simulink model "lab2_aula"  (R2024b)
settings: Solver=VariableStepAuto  StartTime=0.0  StopTime=10000  MaxStep=1  RelTol=1e-3
settings Model: Creator=Diego Regruto  LastModifiedBy=stefa
settings RTWCC: GPUComputeCapability=3.5

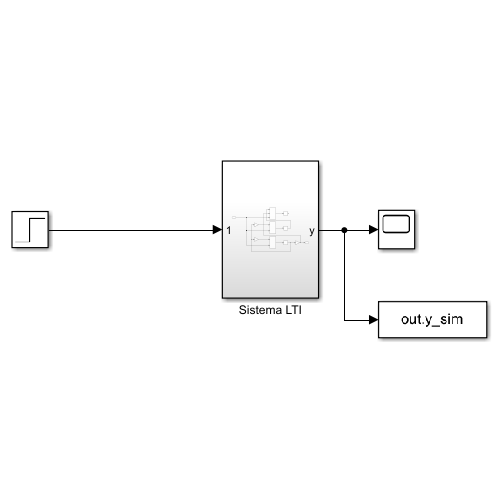
[thumbnail: Simulink's stored preview of the top-level diagram]
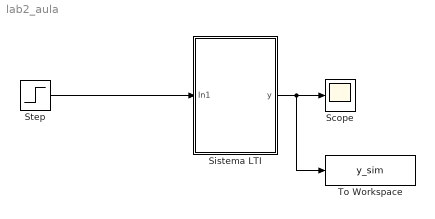
== system lab2_aula ==
  Scope : Scope
  Sistema LTI : Subsystem
  Step : Step  After=9  SampleTime=0
  To Workspace : ToWorkspace  VariableName=y_sim  SaveFormat=Structure With Time  SampleTime=-1
  wires:
  Sistema LTI/1(y) -> To Workspace/1, Scope/1
  Step/1 -> Sistema LTI/1(In1)

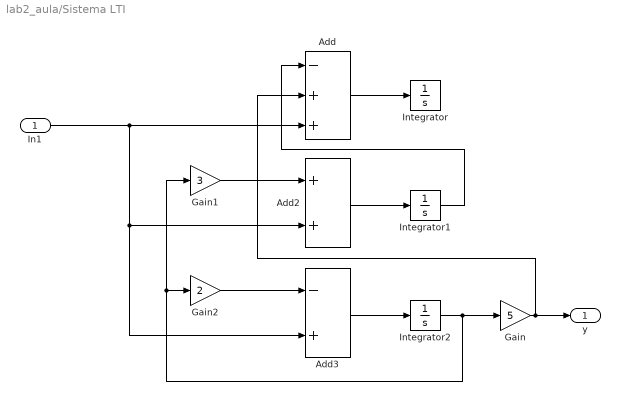
== system lab2_aula/Sistema LTI ==
  In1 : Inport
  Add : Sum  Inputs=-++
  Add2 : Sum
  Add3 : Sum  Inputs=-+
  Gain : Gain  Gain=5
  Gain1 : Gain  Gain=3
  Gain2 : Gain  Gain=2
  Integrator : Integrator  InitialCondition=81
  Integrator1 : Integrator  InitialCondition=15
  Integrator2 : Integrator
  y : Outport
  wires:
  Add3/1 -> Integrator2/1
  Add/1 -> Integrator/1
  Add2/1 -> Integrator1/1
  Gain/1 -> Add/2, y/1
  Integrator2/1 -> Gain2/1, Gain1/1, Gain/1
  Integrator1/1 -> Add/1
  In1/1 -> Add3/2, Add2/2, Add/3
  Gain1/1 -> Add2/1
  Gain2/1 -> Add3/1
